simulink model "motor_sws"  (R2025a)
settings: Solver=FixedStepAuto  StartTime=0  StopTime=5  FixedStep=1e-4  RelTol=1e-3
undefined symbols (not defined in the file): f_supply, fault_severity, Torque_in, V_in
libraries: spsAsynchronousMachineSIUnitsLib x1, spsThreePhaseSourceLib x1, spspowerguiLib x1
settings Model: Creator=User  LastModifiedBy=User
settings DataIOCC: SaveOutput=off  DSMLogging=off  ReturnWorkspaceOutputs=off

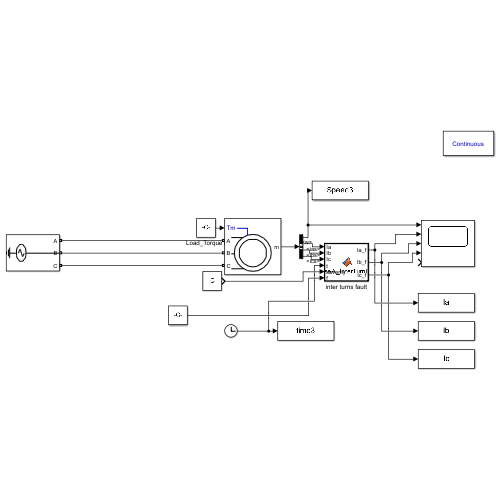
[thumbnail: Simulink's stored preview of the top-level diagram]
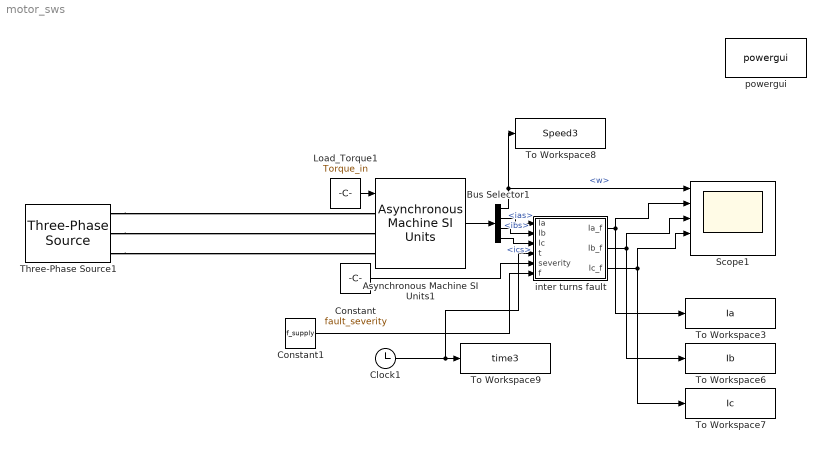
== system motor_sws ==
  Asynchronous Machine SI Units1 : spsAsynchronousMachineSIUnitsLib/Asynchronous Machine SI Units  RotorType=Squirrel-cage  PresetModel=No  MechanicalLoad=Torque Tm  ShowDetailedParameters=on  ReferenceFrame=Stationary  Units=SI  MeasurementBus=on  NominalParameters=[7500 400 50]  VoltageRatio=1  Stator=[1.405 0.005839]  Rotor=[1.395 0.005839]  Cage1=[0.4155 0.002066]  Cage2=[0.4168 0.0003495]  Lm=0.1722  Mechanical=[0.0131 0.001 2]  PolePairs=2  InitialConditions=[0 0 0 0 0 0 0 0]  SimulateSaturation=off  Saturation=[14.03593122, 27.81365428, 53.79336849, 72.68890987, 97.98006896, 148.6815601, 215.7428561, 302.9841135, 428.7778367 ; 230, 322, 414, 460, 506, 552, 598, 644, 690]  LoadFlowParameters=1492000  TsPowergui=0  TsBlock=-1  IterativeModel=Trapezoidal non iterative  IterativeDiscreteModel=Trapezoidal non iterative  Pmec=1.492e+006
  Bus Selector1 : BusSelector  OutputSignals=w,ias,ibs,ics
  Clock1 : Clock
  Constant : Constant  Value=fault_severity
  Constant1 : Constant  Value=f_supply
  Load_Torque1 : Constant  Value=Torque_in
  Scope1 : Scope  NumInputPorts=5
      settings: ActiveDisplayYMinimum=-0.049617664684487431  ActiveDisplayYMaximum=0.049617664684487604
  Three-Phase Source1 : spsThreePhaseSourceLib/Three-Phase Source  InternalConnection=Yg  VoltagePhases=on  Voltage=400  PhaseAngle=0  Voltage_phases=[V_in V_in V_in]/sqrt(3)  PhaseAngles_phases=[0 -120 +120]  Frequency=50  NonIdealSource=off  SpecifyImpedance=off  Resistance=0.8929  Inductance=16.58e-3  ShortCircuitLevel=100e6  BaseVoltage=25e3  XRratio=7  BusType=swing  Pref=10e3  Qref=0  Prefabc=[10e3, 10e3, 10e3]  Qrefabc=[0, 0, 0]  Qmin=-inf  Qmax=inf
  To Workspace3 : ToWorkspace  VariableName=Ia  SampleTime=-1
  To Workspace6 : ToWorkspace  VariableName=Ib  SampleTime=-1
  To Workspace7 : ToWorkspace  VariableName=Ic  SampleTime=-1
  To Workspace8 : ToWorkspace  VariableName=Speed3  SampleTime=-1
  To Workspace9 : ToWorkspace  VariableName=time3  SampleTime=-1
  inter turns fault : MATLAB Function  TreatAsAtomicUnit=on
  powergui : spspowerguiLib/powergui  Priority=1  SimulationMode=Continuous  SampleTime=50e-6  frequency=60  Iterations=50  frequencyindice=50  Pbase=100e6  ErrMax=1e-4  UnitsV=kV  UnitsW=MW  buscounter=0  FunctionMessages=off  echomessages=off  EnableUseOfTLC=off  CurrentSourceSwitches=off  DisableSnubberDevices=off  DisableRonSwitches=off  DisableVfSwitches=off  DisplayEquations=off  AutomaticDiscreteSolvers=off  SolverType=Tustin/Backward Euler (TBE)  Interpol=off  ExternalGateDelay=off  methode=off  Ts=100  x0status=blocks  SPID=on  SwTol=0  HookPort=off  NonlinearTolerance=1e-4  nMaxIteration=100  ContinueOnMaxIteration=off  RestoreLinks=warning  ResistiveCurrentMeasurement=off  Frange=[0:2:500]  Ylog=off  Xlog=on  ShowGrid=off  save=off  variable=ZData  structure=0  ZoomFFT=off  StartTime=0.0  cycles=1  DisplayStyle=1  fundamental=60  FreqAxis=off  MaxFrequency=1000  frequencyindicesteady=1  RmsSteady=1  display=off
  wires:
  Load_Torque1/1 -> Asynchronous Machine SI Units1/1
  Bus Selector1/1 -> To Workspace8/1, Scope1/1  "<w>"
  Asynchronous Machine SI Units1/1 -> Bus Selector1/1
  Clock1/1 -> inter turns fault/4(t), To Workspace9/1
  inter turns fault/3(Ic_f) -> Scope1/4, To Workspace7/1
  inter turns fault/1(Ia_f) -> Scope1/2, To Workspace3/1
  inter turns fault/2(Ib_f) -> Scope1/3, To Workspace6/1
  Bus Selector1/2 -> inter turns fault/1(Ia)  "<ias>"
  Bus Selector1/3 -> inter turns fault/2(Ib)  "<ibs>"
  Bus Selector1/4 -> inter turns fault/3(Ic)  "<ics>"
  Constant/1 -> inter turns fault/5(severity)
  Constant1/1 -> inter turns fault/6(f)
  connections:
  Three-Phase Source1/RConn3 -- Asynchronous Machine SI Units1/LConn3
  Three-Phase Source1/RConn1 -- Asynchronous Machine SI Units1/LConn1
  Three-Phase Source1/RConn2 -- Asynchronous Machine SI Units1/LConn2

== matlab function motor_sws/inter turns fault ==
  data: Ia input; Ia_f output; Ib input; Ic input; t input; Ib_f output; Ic_f output; severity input; f input
function [Ia_f, Ib_f, Ic_f] = PhaseA_InterTurnFault(Ia, Ib, Ic, t, severity, f)
    %#codegen
    % PHASE A INTER-TURN FAULT - Simulink compatible
    % Inputs: Ia, Ib, Ic - phase currents (A)
    %         t - time (s)
    %         severity - 0 to 1 (0=healthy, 1=worst fault)
    % Outputs: Faulty phase currents

    % Fixed parameters
                    % Supply frequency (Hz)
    I_base = 15.3;             % Peak current of healthy motor (A)
    
    % --- FAULT MODEL ---
    
    % 1. Amplitude increase in faulty phase
    % Shorting turns reduces impedance, increasing current
    Ia_increase = 1 + severity * 0.8;
    
    % 2. Fault harmonic components
    % Inter-turn faults create odd harmonics
    if severity > 0
        % Fault signal with decaying effect (simulates arcing)
        tau = 0.1;  % Time constant for fault development
        fault_envelope = 1 - exp(-t/tau);
        
        % Create harmonic-rich fault current
        fault_current = I_base * severity * fault_envelope * (...
            0.6 * sin(2*pi*f*t) + ...          % Fundamental
            0.25 * sin(2*pi*3*f*t - pi/4) + ... % 3rd harmonic
            0.10 * sin(2*pi*5*f*t - pi/3) + ... % 5th harmonic
            0.05 * sin(2*pi*7*f*t));           % 7th harmonic
    else
        fault_current = 0;
        Ia_increase = 1;
    end
    
    % --- APPLY FAULT ---
    
    % Phase A: Increased amplitude + fault harmonics
    Ia_f = Ia * Ia_increase + fault_current;
    
    % Phases B & C: Slight increase due to neutral shift
    unbalance_factor = 1 + severity * 0.1;
    Ib_f = Ib * unbalance_factor;
    Ic_f = Ic * unbalance_factor;
end
